simulink model "Mass_Spring_Damper_System"  (R2019b)
settings: Solver=VariableStepAuto  StartTime=0.0  StopTime=10.0  RelTol=1e-3
values from neighbouring files (symbols this model uses):
  b = 10    [Mass_Spring_Damper_System.m]
  F = 1    [Mass_Spring_Damper_System.m]
  k = 20    [Mass_Spring_Damper_System.m]
  M = 10    [Mass_Spring_Damper_System.m]
settings Model: Creator=Kudi Okerulu  LastModifiedBy=Kudi Okerulu

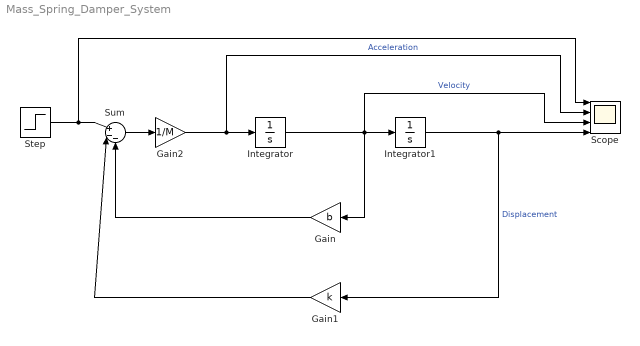
== system Mass_Spring_Damper_System ==
  Gain : Gain  Gain=b
  Gain1 : Gain  Gain=k
  Gain2 : Gain  Gain=1/M
  Integrator : Integrator
  Integrator1 : Integrator
  Scope : Scope  NumInputPorts=4
  Step : Step  After=F  SampleTime=0
  Sum : Sum  Inputs=|+--
  wires:
  Integrator/1 -> Scope/3, Gain/1, Integrator1/1  "Velocity"
  Integrator1/1 -> Scope/4, Gain1/1  "Displacement"
  Sum/1 -> Gain2/1
  Gain/1 -> Sum/3
  Gain1/1 -> Sum/2
  Step/1 -> Scope/1, Sum/1
  Gain2/1 -> Scope/2, Integrator/1  "Acceleration"
